simulink model "SimForcesGP2017a"  (R2020b)
settings: Solver=ode4  StartTime=0.0  StopTime=10  FixedStep=0.001  MaxStep=0.001  RelTol=1e-7
values from neighbouring files (symbols this model uses):
  B11_r_B11C = [0.23805608; 0.13201777; 0]    [InitializeSimulationGP.m]
  B11_r_B11Tc1 = [L11; 0; 0]    [InitializeSimulationGP.m]
  B11_Rot_Tc1 = eye(3)    [InitializeSimulationGP.m]
  B11cI = [0.28426000 -0.06487287 0;         -0.06487287  0.54237481 0;                   0  0          0.67891020]    [InitializeSimulationGP.m]
  B12_r_B12C = [0.60504569; 0.27199376; 0.00002484]    [InitializeSimulationGP.m]
  B12_r_B12Tc2 = [L21;0;0]    [InitializeSimulationGP.m]
  B12_Rot_Tc2 = eye(3)    [InitializeSimulationGP.m]
  B12cI = [1.18803886 -2.36786418 0.00280315;          -2.36786418 6.31493281 0.00022322;           0.00280315 0.00022322 7.40915161]    [InitializeSimulationGP.m]
  B31_r_B31C = [0.35781210 0 0]    [InitializeSimulationGP.m]
  B31_Rot_B41 = eye(3)    [InitializeSimulationGP.m]
  B31cI = diag([0.03150902 0.90735702 0.90763033])    [InitializeSimulationGP.m]
  B32_r_B32C = [0.35781210 0 0]    [InitializeSimulationGP.m]
  B32_Rot_B42 = eye(3)    [InitializeSimulationGP.m]
  B32cI = diag([0.03150902 0.90735702 0.90763033])    [InitializeSimulationGP.m]
  B41_r_B41C = [0.55785997 0 0]    [InitializeSimulationGP.m]
  B41_r_B41Tc1 = [lc1;0;0]    [InitializeSimulationGP.m]
  B41cI = diag([0.00370720 0.55759812 0.55785997])    [InitializeSimulationGP.m]
  B42_r_B42C = [0.55785997 0 0]    [InitializeSimulationGP.m]
  B42_r_B42Tc2 = [lc2; 0; 0]    [InitializeSimulationGP.m]
  B42cI = diag([0.00370720 0.55759812 0.55785997])    [InitializeSimulationGP.m]
  B52_r_B52C = [0 0 0.56802906]    [InitializeSimulationGP.m]
  B52_r_B52P32 = [lc3; 0; 0]    [InitializeSimulationGP.m]
  B52_Rot_P32 = eye(3)    [InitializeSimulationGP.m]
  B52cI = diag([0.91789884, 0.91790043, 0.00091463])    [InitializeSimulationGP.m]
  Bc1_r_Bc1B11 = [L1; 0; 0]    [InitializeSimulationGP.m]
  Bc1_r_Bc1B31 = [0;0;0]    [InitializeSimulationGP.m]
  Bc1_r_Bc1C = [0.14178771; 0.16555780; 0]    [InitializeSimulationGP.m]
  Bc1_V = [0;0;0;0;0;0]    [InitializeSimulationGP.m]
  Bc1cI = [+5.892211080 +5.476111360 -0.000019630;          +5.476111360 +28.66965601 -0.000024550;          -0.000019630 -0.000024550 +29.78955950]    [InitializeSimulationGP.m]
  Bc2_r_Bc2B12 = [L2;0;0]    [InitializeSimulationGP.m]
  Bc2_r_Bc2B32 = [0;0;0]    [InitializeSimulationGP.m]
  Bc2_r_Bc2C = [0.54319901; 0.10543875; 0]    [InitializeSimulationGP.m]
  Bc2cI = [0.48071390 0.52924041 0;          0.52924041 5.80912352 0;              0      0          5.97255351]    [InitializeSimulationGP.m]
  beta1 = atan2d(374.261,935)*pi/180    [InitializeSimulationGP.m]
  beta2 = atan2d(45.757,373.313)*pi/180    [InitializeSimulationGP.m]
  beta3 = atan2d(139.50,1132.19)*pi/180    [InitializeSimulationGP.m]
  beta4 = atan2d(88.061,296.198)*pi/180    [InitializeSimulationGP.m]
  D22F = [0;0;0;0;0;0]    [InitializeSimulationGP.m]
  L1 = 1.0071227324212    (= 1.00712273242)    [InitializeSimulationGP.m]
  L11 = 0.37610632101293    (= 0.376106321013)    [InitializeSimulationGP.m]
  L2 = 1.132185817991    (= 1.13218581799)    [InitializeSimulationGP.m]
  L21 = 0.30901132665325    (= 0.309011326653)    [InitializeSimulationGP.m]
  lc1 = 0.745    [InitializeSimulationGP.m]
  lc2 = 0.745    [InitializeSimulationGP.m]
  mB11 = 25.52660174    [InitializeSimulationGP.m]
  mB12 = 33.92850233    [InitializeSimulationGP.m]
  mB31 = 17.36281648    [InitializeSimulationGP.m]
  mB32 = 17.36281648    [InitializeSimulationGP.m]
  mB41 = 10.34519231    [InitializeSimulationGP.m]
  mB42 = 10.34519231    [InitializeSimulationGP.m]
  mB52 = 6.73059863    [InitializeSimulationGP.m]
  mBc1 = 307.29601379    [InitializeSimulationGP.m]
  mBc2 = 54.58702836    [InitializeSimulationGP.m]
  mP22 = 9.26136143    [InitializeSimulationGP.m]
  mP32 = 570.18877059    [InitializeSimulationGP.m]
  P22_r_P22C = [0.62192523 0 0]    [InitializeSimulationGP.m]
  P22_Rot_B52 = eye(3)    [InitializeSimulationGP.m]
  P22cI = diag([0.00662754, 1.48387017, 1.48398069])    [InitializeSimulationGP.m]
  P32_r_P32C = [0.25466704; -0.13034397; -0.01302248]    [InitializeSimulationGP.m]
  P32_r_P32D22 = [0.40499744871392; -0.13130517281345; -0.013385243295654]    [InitializeSimulationGP.m]
  P32_Rot_D22 = [1 0 0;              0 0.9707729441837 0.23999977258512;              0 -0.23999977258512 0.9707729441837]    [InitializeSimulationGP.m]
  P32cI = [46.81220713 0.38607676 -0.00453819;          0.38607676 71.92201786 -1.14320993;          -0.00453819 -1.14320993 67.38128576]    [InitializeSimulationGP.m]
  Tc1_r_Tc1Bc2 = [0.098495302558553; 0.01838181329939; 0]    [InitializeSimulationGP.m]
  Tc1_Rot_Bc2 = [cos(alpha2) -sin(alpha2) 0;                sin(alpha2)  cos(alpha2) 0;                0            0           1]    [InitializeSimulationGP.m]
  Tc2_r_Tc2P22 = [-0.048858374920227;0.36587359346146;0.035276938723102]    [InitializeSimulationGP.m]
  Tc2_Rot_P22 = [0.95853460763586 -0.27664713597974  0.0683942111482;                0.28497614981675  0.93051946315663 -0.23004808784757;                0                 0.23999977258511  0.9707729441837]    [InitializeSimulationGP.m]
  Th1A = 5*pi/180    (= 0.0872664625997)    [InitializeSimulationGP.m]
  Th1B = 20*pi/180    (= 0.349065850399)    [InitializeSimulationGP.m]
  Th1f = 1    [InitializeSimulationGP.m]
  Th2A = 15*pi/180    (= 0.261799387799)    [InitializeSimulationGP.m]
  Th2B = -50*pi/180    (= -0.872664625997)    [InitializeSimulationGP.m]
  Th2f = 2    [InitializeSimulationGP.m]
  W_r_WBc1 = [0.185;-0.085;0]    [InitializeSimulationGP.m]
  W_Rot_Bc1 = [cos(alpha1) -sin(alpha1) 0;              sin(alpha1)  cos(alpha1) 0;              0            0           1]    [InitializeSimulationGP.m]
  Wg = [0; 9.8066; 0]    [InitializeSimulationGP.m]
  x10 = 0.83    [InitializeSimulationGP.m]
  x20 = 0.83    [InitializeSimulationGP.m]
  xf = [1;0;0;0;0;0]    [InitializeSimulationGP.m]
  xt2A = 0.1    [InitializeSimulationGP.m]
  xt2B = 0.5    [InitializeSimulationGP.m]
  xt2f = 1    [InitializeSimulationGP.m]
  ztau = [0;0;0;0;0;1]    [InitializeSimulationGP.m]
undefined symbols (not defined in the file or in its folder): B11_V, B11_V_SS, B11Ftot, B12_U_Tc2, B12_V, B12_V_SS, B12Ftot, B31_r_B31B41, B31_V, B31_V_SS, B31FTot, B32_r_B32B42, B32_U_B42, B32_V, B32_V_SS, B32FTot, B41_V, B41_V_SS, B41FTot, B42_Rot_Tc2, B42_U_Tc2, B42_V, B42_V_SS, B42FTot, B52_U_P32, B52_V, B52_V_SS, B52Ftot, Bc1_V_SS, Bc1Tot, Bc2_Rot_B12, Bc2_Rot_B32, Bc2_U_B12, Bc2_U_B32, Bc2_V, Bc2_V_SS, Bc2Tot, D22_V, D22_V_SS, dq1, dq11, dq12, dq2, dq21, dq22, dx1, dx2, FTot_S1, FTot_S2P, FTot_S2R, P22_r_P22B52, P22_U_B52, P22_V, P22_V_SS, P22FTot, P32_U_D22, P32_V, P32_V_SS, P32FTot, q1 ... (+28)
libraries: nesl_utility x94, sm_lib x45
(part 3 of 5)

== system SimForcesGP2017a/Hydraulic manipulator, Simscape/TiltCylinderAndTiltPiston ==
  B32Aux : sm_lib/Frames and Transforms/Rigid Transform  TranslationMethod=None  TranslationStandardOffset=0  TranslationLengthUnit=m  TranslationStandardAxis=+Z  TranslationCartesianOffset=[0 0 0]  TranslationROffset=0  TranslationROffsetUnits=m  TranslationZOffset=0  TranslationZOffsetUnits=m  TranslationThetaOffset=0  TranslationThetaOffsetUnits=deg  RotationMethod=StandardAxis  RotationAngleUnits=deg  RotationStandardAxis=+Y  RotationAngle=90  RotationArbitraryAxis=[0 0 1]  FollAlignAxisA=+X  BaseAlignAxisA=+Y  FollAlignAxisB=+Y  BaseAlignAxisB=+Z  RotationSequenceAxes=FollowerAxes  RotationSequence=XYX  RotationSequenceAngles=[0 0 0]  RotationSequenceAnglesUnits=deg  RotationMatrix=[1 0 0; 0 1 0; 0 0 1]
  B42Aux : sm_lib/Frames and Transforms/Rigid Transform  TranslationMethod=None  TranslationStandardOffset=0  TranslationLengthUnit=m  TranslationStandardAxis=+Z  TranslationCartesianOffset=[0 0 0]  TranslationROffset=0  TranslationROffsetUnits=m  TranslationZOffset=0  TranslationZOffsetUnits=m  TranslationThetaOffset=0  TranslationThetaOffsetUnits=deg  RotationMethod=StandardAxis  RotationAngleUnits=deg  RotationStandardAxis=+Y  RotationAngle=-90  RotationArbitraryAxis=[0 0 1]  FollAlignAxisA=+X  BaseAlignAxisA=+Y  FollAlignAxisB=+Y  BaseAlignAxisB=+Z  RotationSequenceAxes=FollowerAxes  RotationSequence=XYX  RotationSequenceAngles=[0 0 0]  RotationSequenceAnglesUnits=deg  RotationMatrix=[1 0 0; 0 1 0; 0 0 1]
  PS-Sim2 : nesl_utility/PS-Simulink Converter  PhysicalDomain=network_engine_domain  SubClassName=ps_output  LeftPortType=input  RightPortType=output  PseudoPeriodic=off  Frequencies=[]  Unit=inherit  AffineConversion=off
  Tilt cylinder rotation (q21) : sm_lib/Joints/Revolute Joint  JointMode=Normal  SenseConstraintForce=off  SenseConstraintForceX=off  SenseConstraintForceY=off  SenseConstraintForceZ=off  SenseConstraintTorque=off  SenseConstraintTorqueX=off  SenseConstraintTorqueY=off  SenseConstraintTorqueZ=off  SenseTotalForce=off  SenseTotalForceX=off  SenseTotalForceY=off  SenseTotalForceZ=off  SenseTotalTorque=off  SenseTotalTorqueX=off  SenseTotalTorqueY=off  SenseTotalTorqueZ=off  CompositeWrenchDir=FollowerOnBase  CompositeWrenchFrame=BaseFrame  EquilibriumPosition=0  EquilibriumPositionUnits=deg  SpringStiffness=0  SpringStiffnessUnits=N*m/deg  DampingCoefficient=0  DampingCoefficientUnits=N*m/(deg/s)  TorqueActuationMode=NoTorque  MotionActuationMode=ComputedMotion  SensePosition=off  SenseVelocity=off  SenseAcceleration=off  SenseTorqueForce=off  SenseLowerLimitTorqueForce=off  SenseUpperLimitTorqueForce=off  LowerLimitSpecify=off  LowerLimitBound=-90  LowerLimitBoundUnits=deg  LowerLimitStiffness=1e4  LowerLimitStiffnessUnits=N*m/deg  LowerLimitDamping=10  LowerLimitDampingUnits=N*m/(deg/s)  LowerLimitTransitionRegionWidth=0.1  LowerLimitTransitionRegionWidthUnits=deg  UpperLimitSpecify=off  UpperLimitBound=90  UpperLimitBoundUnits=deg  UpperLimitStiffness=1e4  UpperLimitStiffnessUnits=N*m/deg  UpperLimitDamping=10  UpperLimitDampingUnits=N*m/(deg/s)  UpperLimitTransitionRegionWidth=0.1  UpperLimitTransitionRegionWidthUnits=deg  PositionTargetSpecify=off  PositionTargetPriority=High  PositionTargetValue=0  PositionTargetValueUnits=deg  VelocityTargetSpecify=off  VelocityTargetPriority=High  VelocityTargetValue=0  VelocityTargetValueUnits=deg/s
  Tilt piston rotation (q22) : sm_lib/Joints/Revolute Joint  JointMode=Normal  SenseConstraintForce=off  SenseConstraintForceX=off  SenseConstraintForceY=off  SenseConstraintForceZ=off  SenseConstraintTorque=off  SenseConstraintTorqueX=off  SenseConstraintTorqueY=off  SenseConstraintTorqueZ=off  SenseTotalForce=off  SenseTotalForceX=off  SenseTotalForceY=off  SenseTotalForceZ=off  SenseTotalTorque=off  SenseTotalTorqueX=off  SenseTotalTorqueY=off  SenseTotalTorqueZ=off  CompositeWrenchDir=FollowerOnBase  CompositeWrenchFrame=BaseFrame  EquilibriumPosition=0  EquilibriumPositionUnits=deg  SpringStiffness=0  SpringStiffnessUnits=N*m/deg  DampingCoefficient=0  DampingCoefficientUnits=N*m/(deg/s)  TorqueActuationMode=NoTorque  MotionActuationMode=ComputedMotion  SensePosition=off  SenseVelocity=off  SenseAcceleration=off  SenseTorqueForce=off  SenseLowerLimitTorqueForce=off  SenseUpperLimitTorqueForce=off  LowerLimitSpecify=off  LowerLimitBound=-90  LowerLimitBoundUnits=deg  LowerLimitStiffness=1e4  LowerLimitStiffnessUnits=N*m/deg  LowerLimitDamping=10  LowerLimitDampingUnits=N*m/(deg/s)  LowerLimitTransitionRegionWidth=0.1  LowerLimitTransitionRegionWidthUnits=deg  UpperLimitSpecify=off  UpperLimitBound=90  UpperLimitBoundUnits=deg  UpperLimitStiffness=1e4  UpperLimitStiffnessUnits=N*m/deg  UpperLimitDamping=10  UpperLimitDampingUnits=N*m/(deg/s)  UpperLimitTransitionRegionWidth=0.1  UpperLimitTransitionRegionWidthUnits=deg  PositionTargetSpecify=off  PositionTargetPriority=High  PositionTargetValue=0  PositionTargetValueUnits=deg  VelocityTargetSpecify=off  VelocityTargetPriority=High  VelocityTargetValue=0  VelocityTargetValueUnits=deg/s
  TiltCylinderSolid : sm_lib/Body Elements/File Solid  ExtGeomFileName=05_TiltCylGP.STEP  UnitType=FromFile  ExtGeomFileUnits=m  StepReaderType=OCC  ExportConvexHullGeometry=off  InertiaType=Custom  Mass=17.36281648  MassUnits=kg  CenterOfMass=[0 0.31781210 0]  CenterOfMassUnits=m  MomentsOfInertia=[0.90735702 0.03150902 0.90763033]  MomentsOfInertiaUnits=kg*m^2  ProductsOfInertia=[0 0 0]  ProductsOfInertiaUnits=kg*m^2  BasedOnType=Density  Density=7300  DensityUnits=kg/m^3  DoExposeReferenceFrame=off  SerializedFrames=<Frames><Frame><Id>Frame1</Id><Value><Name>B32</Name><Origin><Source>GeometricFeature</Source><FeatureName>cylindrical surface 11</FeatureName></Origin><PrimaryAxis><DefinedDirection>+X</DefinedDirection><Source>ReferenceFrame</Source><SourceDirection>+Y</SourceDirection><FeatureName></FeatureName></PrimaryAxis><SecondaryAxis><DefinedDirection>+Y</DefinedDirection><Source>ReferenceFrame</Source><SourceDirection>-X</SourceDirection><FeatureName></FeatureName></SecondaryAxis></Value></Frame><Frame><Id>Frame2</Id><Value><Name>B32Aux</Name><Origin><Source>GeometricFeature</Source><FeatureName>planar surface 4</FeatureName></Origin><PrimaryAxis><DefinedDirection>+X</DefinedDirection><Source>ReferenceFrame</Source><SourceDirection>+Y</SourceDirection><FeatureName></FeatureName></PrimaryAxis><SecondaryAxis><DefinedDirection>+Y</DefinedDirection><Source>ReferenceFrame</Source><SourceDirection>-X</SourceDirection><FeatureName></FeatureName></SecondaryAxis></Value></Frame></Frames>  GraphicType=FromGeometry  MarkerShape=Sphere  MarkerSize=10  GraphicVisPropType=SimpleVisualProperties  GraphicDiffuseColor=[1 1 119]/255  GraphicSpecularColor=[0.5 0.5 0.5 1.0]  GraphicAmbientColor=[0.15 0.15 0.15 1.0]  GraphicEmissiveColor=[0.0 0.0 0.0 1.0]  GraphicShininess=75  GraphicOpacity=1.0
  TiltPistonSolid : sm_lib/Body Elements/File Solid  ExtGeomFileName=06_TiltPistGP.STEP  UnitType=FromFile  ExtGeomFileUnits=m  StepReaderType=OCC  ExportConvexHullGeometry=off  InertiaType=Custom  Mass=10.34519231  MassUnits=kg  CenterOfMass=[0 0.32981882 0]  CenterOfMassUnits=m  MomentsOfInertia=[0.55759812 0.00370720 0.55785997]  MomentsOfInertiaUnits=kg*m^2  ProductsOfInertia=[0 0 0]  ProductsOfInertiaUnits=kg*m^2  BasedOnType=Density  Density=7850  DensityUnits=kg/m^3  DoExposeReferenceFrame=off  SerializedFrames=<Frames><Frame><Id>Frame2</Id><Value><Name>B42</Name><Origin><Source>GeometricFeature</Source><FeatureName>planar surface 2</FeatureName></Origin><PrimaryAxis><DefinedDirection>+X</DefinedDirection><Source>ReferenceFrame</Source><SourceDirection>+Y</SourceDirection><FeatureName></FeatureName></PrimaryAxis><SecondaryAxis><DefinedDirection>+Y</DefinedDirection><Source>ReferenceFrame</Source><SourceDirection>-X</SourceDirection><FeatureName></FeatureName></SecondaryAxis></Value></Frame><Frame><Id>Frame3</Id><Value><Name>P11</Name><Origin><Source>GeometricFeature</Source><FeatureName>cylindrical surface 8</FeatureName></Origin><PrimaryAxis><DefinedDirection>+X</DefinedDirection><Source>ReferenceFrame</Source><SourceDirection>+Y</SourceDirection><FeatureName></FeatureName></PrimaryAxis><SecondaryAxis><DefinedDirection>+Y</DefinedDirection><Source>ReferenceFrame</Source><SourceDirection>-X</SourceDirection><FeatureName></FeatureName></SecondaryAxis></Value></Frame></Frames>  GraphicType=FromGeometry  MarkerShape=Sphere  MarkerSize=10  GraphicVisPropType=SimpleVisualProperties  GraphicDiffuseColor=[9 232 232]/255  GraphicSpecularColor=[0.5 0.5 0.5 1.0]  GraphicAmbientColor=[0.15 0.15 0.15 1.0]  GraphicEmissiveColor=[0.0 0.0 0.0 1.0]  GraphicShininess=75  GraphicOpacity=1.0
  x2-translation : sm_lib/Joints/Prismatic Joint  JointMode=Normal  SenseConstraintForce=off  SenseConstraintForceX=off  SenseConstraintForceY=off  SenseConstraintForceZ=off  SenseConstraintTorque=off  SenseConstraintTorqueX=off  SenseConstraintTorqueY=off  SenseConstraintTorqueZ=off  SenseTotalForce=off  SenseTotalForceX=off  SenseTotalForceY=off  SenseTotalForceZ=off  SenseTotalTorque=off  SenseTotalTorqueX=off  SenseTotalTorqueY=off  SenseTotalTorqueZ=off  CompositeWrenchDir=FollowerOnBase  CompositeWrenchFrame=FollowerFrame  EquilibriumPosition=0  EquilibriumPositionUnits=m  SpringStiffness=0  SpringStiffnessUnits=N/m  DampingCoefficient=0  DampingCoefficientUnits=N/(m/s)  TorqueActuationMode=ComputedTorque  MotionActuationMode=ComputedMotion  SensePosition=off  SenseVelocity=off  SenseAcceleration=off  SenseTorqueForce=on  SenseLowerLimitTorqueForce=off  SenseUpperLimitTorqueForce=off  LowerLimitSpecify=off  LowerLimitBound=-1  LowerLimitBoundUnits=m  LowerLimitStiffness=1e6  LowerLimitStiffnessUnits=N/m  LowerLimitDamping=1e3  LowerLimitDampingUnits=N/(m/s)  LowerLimitTransitionRegionWidth=1e-4  LowerLimitTransitionRegionWidthUnits=m  UpperLimitSpecify=off  UpperLimitBound=1  UpperLimitBoundUnits=m  UpperLimitStiffness=1e6  UpperLimitStiffnessUnits=N/m  UpperLimitDamping=1e3  UpperLimitDampingUnits=N/(m/s)  UpperLimitTransitionRegionWidth=1e-4  UpperLimitTransitionRegionWidthUnits=m  PositionTargetSpecify=on  PositionTargetPriority=Low  PositionTargetValue=0.4  PositionTargetValueUnits=m  VelocityTargetSpecify=off  VelocityTargetPriority=High  VelocityTargetValue=0  VelocityTargetValueUnits=m/s
  B32 : PMIOPort  Side=Left
  B42 : PMIOPort  Port=2  Side=Left
  F4 : PMIOPort  Port=3  Side=Right
  F6 : PMIOPort  Port=4  Side=Right
  fc2 : Outport
  wires:
  PS-Sim2/1 -> fc2/1
  connections:
  TiltCylinderSolid/RConn1 -- B32Aux/LConn1
  x2-translation/RConn1 -- B42Aux/LConn1
  Tilt cylinder rotation (q21)/RConn1 -- TiltCylinderSolid/LConn1 -- B32/RConn1
  B42/RConn1 -- TiltPistonSolid/LConn1 -- B42Aux/RConn1
  B32Aux/RConn1 -- x2-translation/LConn1
  Tilt cylinder rotation (q21)/LConn1 -- F4/RConn1
  TiltPistonSolid/RConn1 -- Tilt piston rotation (q22)/LConn1
  Tilt piston rotation (q22)/RConn1 -- F6/RConn1
  PS-Sim2/LConn1 -- x2-translation/RConn2

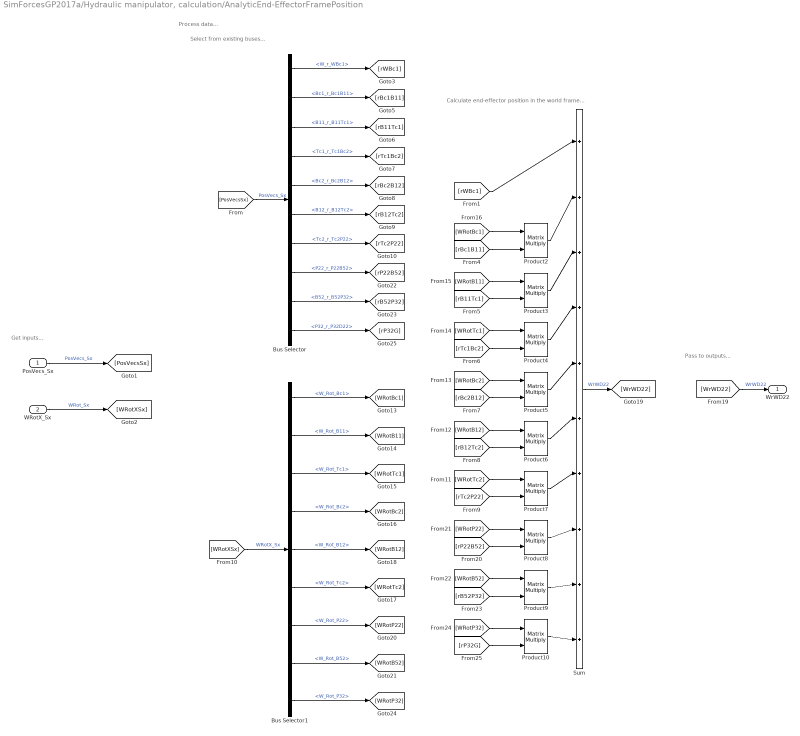
== system SimForcesGP2017a/Hydraulic manipulator, calculation/AnalyticEnd-EffectorFramePosition ==
  note: Pass to outputs...
  note: Process data...
  note: Select from existing buses...
  note: Calculate end-effector position in the world frame...
  note: Get inputs...
  PosVecs_Sx : Inport
  WRotX_Sx : Inport  Port=2
  Bus Selector : BusSelector  OutputSignals=PosVecs_S1.W_r_WBc1,PosVecs_S1.Bc1_r_Bc1B11,PosVecs_S1.B11_r_B11Tc1,PosVecs_S1.Tc1_r_Tc1Bc2,PosVecs_S2R.Bc2_r_Bc2B12,PosVecs_S2R.B12_r_B12Tc2,PosVecs_S2R.Tc2_r_Tc2P22,PosVecs_S2P.P22_r_P22B52,PosVecs_S2P.B52_r_B52P32,PosVecs_S2P.P32_r_P32D22
  Bus Selector1 : BusSelector  OutputSignals=WRotX_S1.W_Rot_Bc1,WRotX_S1.W_Rot_B11,WRotX_S1.W_Rot_Tc1,WRotX_S1.W_Rot_Bc2,WRotX_S2R.W_Rot_B12,WRotX_S2R.W_Rot_Tc2,WRotX_S2R.W_Rot_P22,WRotX_S2P.W_Rot_B52,WRotX_S2P.W_Rot_P32
  Product{2..10} (9 alike) : Product  Multiplication=Matrix(*)
  Sum : Sum  Inputs=|++++++++++
  WrWD22 : Outport
  wires:
  WRotX_Sx/1 -> [WRotXSx]  "WRot_Sx"
  PosVecs_Sx/1 -> [PosVecsSx]  "PosVecs_Sx"
  [PosVecsSx] -> Bus Selector/1  "PosVecs_Sx"
  Bus Selector/2 -> [rBc1B11]  "<Bc1_r_Bc1B11>"
  Bus Selector/3 -> [rB11Tc1]  "<B11_r_B11Tc1>"
  Bus Selector/7 -> [rTc2P22]  "<Tc2_r_Tc2P22>"
  Bus Selector/6 -> [rB12Tc2]  "<B12_r_B12Tc2>"
  Bus Selector/5 -> [rBc2B12]  "<Bc2_r_Bc2B12>"
  Bus Selector/4 -> [rTc1Bc2]  "<Tc1_r_Tc1Bc2>"
  [rBc1B11] -> Product2/2
  [rB11Tc1] -> Product3/2
  [rTc1Bc2] -> Product4/2
  [rBc2B12] -> Product5/2
  [rB12Tc2] -> Product6/2
  [rTc2P22] -> Product7/2
  [WRotXSx] -> Bus Selector1/1  "WRotX_Sx"
  Bus Selector1/1 -> [WRotBc1]  "<W_Rot_Bc1>"
  Bus Selector1/2 -> [WRotB11]  "<W_Rot_B11>"
  Bus Selector1/3 -> [WRotTc1]  "<W_Rot_Tc1>"
  Bus Selector1/4 -> [WRotBc2]  "<W_Rot_Bc2>"
  Bus Selector1/5 -> [WRotB12]  "<W_Rot_B12>"
  Bus Selector1/6 -> [WRotTc2]  "<W_Rot_Tc2>"
  [WRotTc2] -> Product7/1
  [WRotB12] -> Product6/1
  [WRotBc2] -> Product5/1
  [WRotTc1] -> Product4/1
  [WRotB11] -> Product3/1
  [WRotBc1] -> Product2/1
  Sum/1 -> [WrWD22]  "WrWD22"
  [WrWD22] -> WrWD22/1  "WrWD22"
  Bus Selector1/7 -> [WRotP22]  "<W_Rot_P22>"
  Bus Selector1/8 -> [WRotB52]  "<W_Rot_B52>"
  Bus Selector/8 -> [rP22B52]  "<P22_r_P22B52>"
  Bus Selector/9 -> [rB52P32]  "<B52_r_B52P32>"
  [rP22B52] -> Product8/2
  [WRotP22] -> Product8/1
  [WRotB52] -> Product9/1
  [rB52P32] -> Product9/2
  Bus Selector1/9 -> [WRotP32]  "<W_Rot_P32>"
  Bus Selector/10 -> [rP32G]  "<P32_r_P32D22>"
  [rP32G] -> Product10/2
  [WRotP32] -> Product10/1
  Bus Selector/1 -> [rWBc1]  "<W_r_WBc1>"
  [rWBc1] -> Sum/1
  Product2/1 -> Sum/2
  Product3/1 -> Sum/3
  Product4/1 -> Sum/4
  Product5/1 -> Sum/5
  Product6/1 -> Sum/6
  Product7/1 -> Sum/7
  Product8/1 -> Sum/8
  Product9/1 -> Sum/9
  Product10/1 -> Sum/10

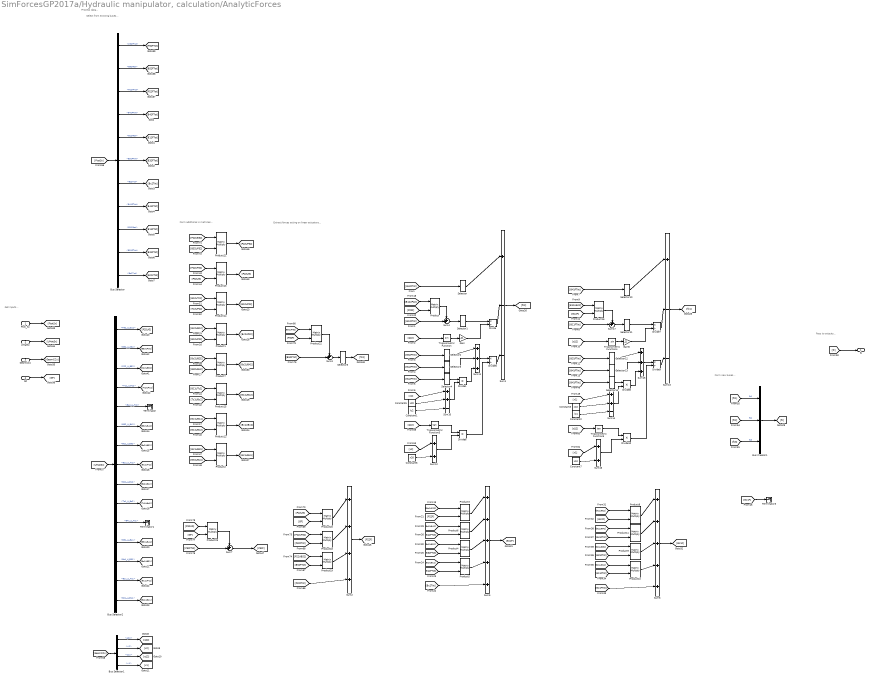
== system SimForcesGP2017a/Hydraulic manipulator, calculation/AnalyticForces ==
  note: Pass to outputs...
  note: Form new buses...
  note: Process data...
  note: Extract forces acting on linear actuators...
  note: Form additional U matrices...
  note: Select from existing buses...
  note: Get inputs...
  Ftot_Sx : Inport
  UMatSx : Inport  Port=2
  GeomCCx : Inport  Port=3
  GF : Inport  Port=4
  Bus Creator1 : BusCreator  Inputs=3
  Bus Selector : BusSelector  OutputSignals=FTot_S2P.P32FTot,FTot_S2P.B52Ftot,FTot_S2P.P22FTot,FTot_S2R.B42FTot,FTot_S2R.B12Ftot,FTot_S2R.B32FTot,FTot_S2R.Bc2Tot,FTot_S1.B41FTot,FTot_S1.B11Ftot,FTot_S1.B31FTot,FTot_S1.Bc1Tot
  Bus Selector1 : BusSelector  OutputSignals=Geom_S2R.q22,Geom_S2R.x2,Geom_S1.q12,Geom_S1.x1
  Bus Selector2 : BusSelector  OutputSignals=UMats_S2P.P32_U_D22,UMats_S2P.B52_U_P32,UMats_S2P.P22_U_B52,UMats_S2R.Tc2_U_P22,UMats_S2R.B42_U_Tc2,UMats_S2R.B32_U_B42,UMats_S2R.Bc2_U_B32,UMats_S2R.B12_U_Tc2,UMats_S2R.Bc2_U_B12,UMats_S1.Tc1_U_Bc2,UMats_S1.B41_U_Tc1,UMats_S1.B31_U_B41,UMats_S1.Bc1_U_B31,UMats_S1.B11_U_Tc1,UMats_S1.Bc1_U_B11
  Constant1 : Constant  Value=lc2
  Constant2 : Constant  Value=lc1
  Constant3 : Constant  Value=x10
  Constant5 : Constant  Value=x20
  Constant6 : Constant  Value=x20
  Constant7 : Constant  Value=x10
  Divide{,5,7,9} (4 alike) : Product  Inputs=*/
  Divide{1,6,8,10} (4 alike) : Product  Inputs=**
  Gain : Gain  Gain=L21
  Gain5 : Gain  Gain=L11
  Product{,1..16,18..23} (23 alike) : Product  Multiplication=Matrix(*)
  Selector : Selector  InputPortWidth=6  IndexOptions=Index vector (dialog)  Indices=[1]  OutputSizes=1
  Selector{1..3,11..13} (6 alike) : Selector  InputPortWidth=6  IndexOptions=Index vector (dialog)  Indices=[6]  OutputSizes=1
  Selector10 : Selector  InputPortWidth=6  IndexOptions=Index vector (dialog)  Indices=[1]  OutputSizes=1
  Selector14 : Selector  InputPortWidth=6  IndexOptions=Index vector (dialog)  Indices=[2]  OutputSizes=1
  Selector4 : Selector  InputPortWidth=6  IndexOptions=Index vector (dialog)  Indices=[2]  OutputSizes=1
  Selector5 : Selector  InputPortWidth=6  IndexOptions=Index vector (dialog)  Indices=[1]  OutputSizes=1
  Sum1 : Sum  Inputs=|+--
  Sum10 : Sum  Inputs=|++-
  Sum11 : Sum  Inputs=|+++
  Sum12 : Sum  Inputs=|++
  Sum13 : Sum  Inputs=|+--
  Sum14 : Sum  Inputs=|++-
  Sum15 : Sum  Inputs=|+++
  Sum16 : Sum  Inputs=|++
  Sum{3..4,7,17} (4 alike) : Sum  Inputs=++|
  Sum2 : Sum  Inputs=|++++
  Sum5 : Sum  Inputs=|+++++
  Sum6 : Sum  Inputs=|+++++
  Terminator : Terminator
  Terminator1 : Terminator
  Terminator3 : Terminator
  Trigonometric Function : Trigonometry
  Trigonometric Function3 : Trigonometry  Operator=tan
  Trigonometric Function4 : Trigonometry
  Trigonometric Function5 : Trigonometry  Operator=tan
  fc : Outport
  wires:
  Bus Selector/4 -> [B42FTot]  "<B42FTot>"
  Bus Selector/6 -> [B32FTot]  "<B32FTot>"
  Bus Selector/5 -> [B12FTot]  "<B12Ftot>"
  Bus Selector/7 -> [Bc2Tot]  "<Bc2Tot>"
  Bus Selector/8 -> [B41FTot]  "<B41FTot>"
  Bus Selector/9 -> [B11FTot]  "<B11Ftot>"
  Bus Selector/10 -> [B31FTot]  "<B31FTot>"
  Bus Selector/11 -> [Bc1FTot]  "<Bc1Tot>"
  [B42FTot] -> Selector/1
  Bus Selector1/1 -> [q22]  "<q22>"
  Bus Selector1/2 -> [x2]  "<x2>"
  Bus Selector1/4 -> [x1]  "<x1>"
  Bus Selector1/3 -> [q12]  "<q12>"
  Gain/1 -> Divide/2
  Trigonometric Function/1 -> Gain/1
  Selector/1 -> Sum1/1
  Divide/1 -> Sum1/2
  Sum1/1 -> [fc2]
  Bus Selector2/4 -> [Tc2UP22]  "<Tc2_U_P22>"
  Bus Selector2/5 -> Terminator/1  "<B42_U_Tc2>"
  Bus Selector2/6 -> [B32UB42]  "<B32_U_B42>"
  Bus Selector2/7 -> [Bc2UB32]  "<Bc2_U_B32>"
  Bus Selector2/8 -> [B12UTc2]  "<B12_U_Tc2>"
  Bus Selector2/9 -> [Bc2UB12]  "<Bc2_U_B12>"
  Bus Selector2/10 -> [Tc1UBc2]  "<Tc1_U_Bc2>"
  Bus Selector2/11 -> Terminator1/1  "<B41_U_Tc1>"
  Bus Selector2/12 -> [B31UB41]  "<B31_U_B41>"
  Bus Selector2/13 -> [Bc1UB31]  "<Bc1_U_B31>"
  Bus Selector2/14 -> [B11UTc1]  "<B11_U_Tc1>"
  Bus Selector2/15 -> [Bc1UB11]  "<Bc1_U_B11>"
  [B12FTot] -> Sum4/2
  Product/1 -> Sum4/1
  Sum4/1 -> Selector1/1
  [B12UP22] -> Product/1
  [Bc2UP22] -> Product3/1
  [P22F] -> Product/2
  [P22F] -> Product3/2
  Product3/1 -> Sum5/1
  [Bc2Tot] -> Sum5/5
  Product6/1 -> Sum5/2
  Product4/1 -> Sum5/3
  Product5/1 -> Sum5/4
  [B12FTot] -> Product5/2
  [Bc2UB12] -> Product5/1
  [B32FTot] -> Product4/2
  [B42FTot] -> Product6/2
  [B32UB42] -> Product7/2
  [Bc2UB32] -> Product7/1
  Product7/1 -> [Bc2UB42]
  [Bc2UB42] -> Product6/1
  [Bc2UB32] -> Product4/1
  Sum5/1 -> [Bc2F]
  Sum6/1 -> [Bc1F]
  [Bc1UB31] -> Product9/1
  [Bc1UB41] -> Product11/1
  [B41FTot] -> Product11/2
  [B31FTot] -> Product9/2
  [Bc1UB11] -> Product10/1
  [B11FTot] -> Product10/2
  Product10/1 -> Sum6/4
  Product9/1 -> Sum6/3
  Product11/1 -> Sum6/2
  [Bc1FTot] -> Sum6/5
  Product8/1 -> Sum6/1
  [Bc2F] -> Product8/2
  [Bc1UBc2] -> Product8/1
  Product1/1 -> [Bc2UP22]
  Product2/1 -> [Bc1UB41]
  [Bc1UB31] -> Product2/1
  [B31UB41] -> Product2/2
  [B12UTc2] -> Product14/1
  [Tc2UP22] -> Product14/2
  Product14/1 -> [B12UP22]
  [B12UP22] -> Product1/2
  [Bc2UB12] -> Product1/1
  [Bc1UB11] -> Product12/1
  [B11UBc2] -> Product12/2
  Product15/1 -> [B11UBc2]
  [Tc1UBc2] -> Product15/2
  [B11UTc1] -> Product15/1
  Product12/1 -> [Bc1UBc2]
  Selector1/1 -> Divide/1
  Divide5/1 -> Sum1/3
  Constant6/1 -> Sum12/2
  [x2] -> Sum12/1
  Selector2/1 -> Sum11/1
  Selector3/1 -> Sum11/2
  Divide1/1 -> Sum11/3
  [B32FTot] -> Selector2/1
  [B42FTot] -> Selector3/1
  [B42FTot] -> Selector4/1
  Selector4/1 -> Divide1/1
  Sum10/1 -> Divide1/2
  Constant1/1 -> Sum10/3
  [x2] -> Sum10/1
  Constant5/1 -> Sum10/2
  [fc1] -> Bus Creator1/1  "fc1"
  [fc2] -> Bus Creator1/2  "fc2"
  [q22] -> Trigonometric Function/1
  Ftot_Sx/1 -> [FtotSx]
  UMatSx/1 -> [UMatSx]
  GeomCCx/1 -> [GeomCCx]
  GF/1 -> [GF]
  [FtotSx] -> Bus Selector/1
  [UMatSx] -> Bus Selector2/1
  [GeomCCx] -> Bus Selector1/1
  Trigonometric Function3/1 -> Divide6/1
  Sum12/1 -> Divide6/2
  Sum11/1 -> Divide5/1
  Divide6/1 -> Divide5/2
  [q22] -> Trigonometric Function3/1
  [q12] -> Trigonometric Function5/1
  Divide10/1 -> Divide9/2
  Sum15/1 -> Divide9/1
  Sum16/1 -> Divide10/2
  Trigonometric Function5/1 -> Divide10/1
  [q12] -> Trigonometric Function4/1
  Constant3/1 -> Sum14/2
  [x1] -> Sum14/1
  Constant2/1 -> Sum14/3
  Sum14/1 -> Divide8/2
  Selector14/1 -> Divide8/1
  [B41FTot] -> Selector14/1
  [B41FTot] -> Selector13/1
  [B31FTot] -> Selector12/1
  Divide8/1 -> Sum15/3
  Selector13/1 -> Sum15/2
  Selector12/1 -> Sum15/1
  [x1] -> Sum16/1
  Constant7/1 -> Sum16/2
  Divide9/1 -> Sum13/3
  Selector11/1 -> Divide7/1
  [Bc2F] -> Product16/2
  [B11UBc2] -> Product16/1
  Sum17/1 -> Selector11/1
  Product16/1 -> Sum17/1
  [B11FTot] -> Sum17/2
  Sum13/1 -> [fc1]
  Divide7/1 -> Sum13/2
  Selector10/1 -> Sum13/1
  Trigonometric Function4/1 -> Gain5/1
  Gain5/1 -> Divide7/2
  [B41FTot] -> Selector10/1
  Bus Creator1/1 -> [fc]
  [fc] -> fc/1
  Bus Selector/3 -> [P22FTot]  "<P22FTot>"
  Bus Selector/2 -> [B52FTot]  "<B52Ftot>"
  Bus Selector/1 -> [P32FTot]  "<P32FTot>"
  Bus Selector2/1 -> [P32UG]  "<P32_U_D22>"
  Bus Selector2/3 -> [P22UB52]  "<P22_U_B52>"
  Bus Selector2/2 -> [B52UP32]  "<B52_U_P32>"
  Sum2/1 -> [P22F]
  Product18/1 -> Sum2/2
  [P22FTot] -> Sum2/4
  Product19/1 -> Sum2/3
  Product20/1 -> Sum2/1
  [B52FTot] -> Product19/2
  [P32FTot] -> Product18/2
  [GF] -> Product20/2
  [P22UG] -> Product20/1
  [P22UB52] -> Product21/1
  [B52UP32] -> Product21/2
  Product21/1 -> [P22UP32]
  [P22UP32] -> Product18/1
  [P22UB52] -> Product19/1
  [B52FTot] -> Sum3/2
  Product22/1 -> Sum3/1
  [P32FTot] -> Sum7/2
  [GF] -> Product23/2
  [P32UG] -> Product23/1
  Product23/1 -> Sum7/1
  Sum7/1 -> [P32F]
  [P32F] -> Product22/2
  [B52UP32] -> Product22/1
  Sum3/1 -> Selector5/1
  Selector5/1 -> [fc3]
  [fc3] -> Bus Creator1/3  "fc3"
  [Bc1F] -> Terminator3/1
  Product13/1 -> [P22UG]
  [P32UG] -> Product13/2
  [P22UP32] -> Product13/1

== system SimForcesGP2017a/Hydraulic manipulator, calculation/AnalyticTotalForces ==
  note: Process data...
  note: Pass to outputs...
  note: Get inputs...
  Vels_Sx : Inport
  WRotX_Sx : Inport  Port=2
  Bus Creator : BusCreator  Inputs=FTot_S1,FTot_S2R,FTot_S2P
  Structure 1 : Subsystem
  Structure 2 (Prismatic segment) : Subsystem
  Structure 2 (Revolute segment) : Subsystem
  FTot_Sx : Outport
  wires:
  Vels_Sx/1 -> [VelsSx]
  WRotX_Sx/1 -> [WRotSx]
  [VelsSx] -> Structure 1/1(Vels_Sx)
  [VelsSx] -> Structure 2 (Revolute segment)/1(Vels_Sx)
  [WRotSx] -> Structure 1/2(WRotX_Sx)
  [WRotSx] -> Structure 2 (Revolute segment)/2(WRotX_Sx)
  Structure 2 (Revolute segment)/1(FTot_S2R) -> [FTotS2R]
  Structure 1/1(FTot_S1) -> [FTotS1]
  [FTotS2R] -> Bus Creator/2  "FTot_S2R"
  [FTotS1] -> Bus Creator/1  "FTot_S1"
  [FTotSx] -> FTot_Sx/1  "FTot_Sx"
  Bus Creator/1 -> [FTotSx]
  [WRotSx] -> Structure 2 (Prismatic segment)/2(WRotX_Sx)
  [VelsSx] -> Structure 2 (Prismatic segment)/1(Vels_Sx)
  Structure 2 (Prismatic segment)/1(FTot_S2P) -> [FTotS2P]
  [FTotS2P] -> Bus Creator/3  "FTot_S2P"

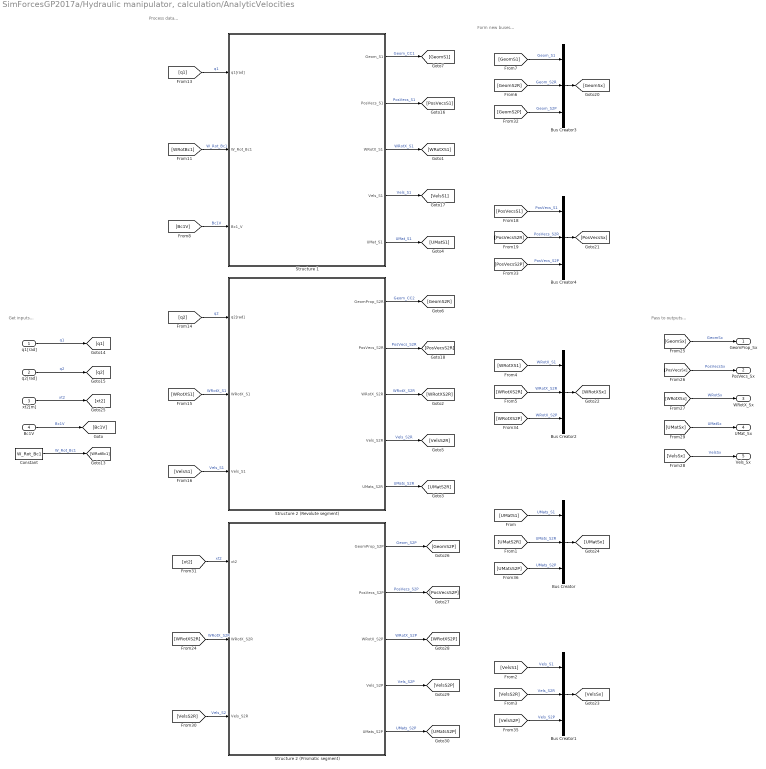
== system SimForcesGP2017a/Hydraulic manipulator, calculation/AnalyticVelocities ==
  note: Pass to outputs...
  note: Form new buses...
  note: Process data...
  note: Get inputs...
  q1[rad] : Inport  Unit=rad
  q2[rad] : Inport  Port=2
  xt2[m] : Inport  Port=3
  Bc1V : Inport  Port=4
  Bus Creator{,1..4} (5 alike) : BusCreator  Inputs=3
  Constant : Constant  Value=W_Rot_Bc1
  Structure 1 : Subsystem
  Structure 2 (Prismatic segment) : Subsystem
  Structure 2 (Revolute segment) : Subsystem
  GeomProp_Sx : Outport
  PosVecs_Sx : Outport  Port=2
  WRotX_Sx : Outport  Port=3
  UMat_Sx : Outport  Port=4
  Vels_Sx : Outport  Port=5
  wires:
  Structure 1/4(Vels_S1) -> [VelsS1]  "Vels_S1"
  [VelsS1] -> Structure 2 (Revolute segment)/3(Vels_S1)  "Vels_S1"
  Structure 2 (Revolute segment)/4(Vels_S2R) -> [VelsS2R]  "Vels_S2R"
  Structure 2 (Revolute segment)/5(UMats_S2R) -> [UMatS2R]  "UMats_S2R"
  Structure 1/5(UMat_S1) -> [UMatS1]  "UMat_S1"
  Structure 1/3(WRotX_S1) -> [WRotXS1]  "WRotX_S1"
  [WRotXS1] -> Structure 2 (Revolute segment)/2(WRotX_S1)  "WRotX_S1"
  Structure 2 (Revolute segment)/3(WRotX_S2R) -> [WRotXS2R]  "WRotX_S2R"
  Structure 2 (Revolute segment)/1(GeomProp_S2R) -> [GeomS2R]  "Geom_CC2"
  Structure 1/1(Geom_S1) -> [GeomS1]  "Geom_CC1"
  Constant/1 -> [WRotBc1]  "W_Rot_Bc1"
  [WRotBc1] -> Structure 1/2(W_Rot_Bc1)  "W_Rot_Bc1"
  [Bc1V] -> Structure 1/3(Bc1_V)  "Bc1V"
  q1[rad]/1 -> [q1]  "q1"
  [q1] -> Structure 1/1(q1[rad])  "q1"
  q2[rad]/1 -> [q2]  "q2"
  [q2] -> Structure 2 (Revolute segment)/1(q2[rad])  "q2"
  Structure 1/2(PosVecs_S1) -> [PosVecsS1]  "PosVecs_S1"
  [PosVecsS1] -> Bus Creator4/1  "PosVecs_S1"
  Structure 2 (Revolute segment)/2(PosVecs_S2R) -> [PosVecsS2R]  "PosVecs_S2R"
  [PosVecsS2R] -> Bus Creator4/2  "PosVecs_S2R"
  [WRotXS2R] -> Bus Creator2/2  "WRotX_S2R"
  [WRotXS1] -> Bus Creator2/1  "WRotX_S1"
  [UMatS2R] -> Bus Creator/2  "UMats_S2R"
  [UMatS1] -> Bus Creator/1  "UMats_S1"
  [VelsS1] -> Bus Creator1/1  "Vels_S1"
  [VelsS2R] -> Bus Creator1/2  "Vels_S2R"
  [GeomS2R] -> Bus Creator3/2  "Geom_S2R"
  [GeomS1] -> Bus Creator3/1  "Geom_S1"
  Bus Creator3/1 -> [GeomSx]
  Bus Creator4/1 -> [PosVecsSx]
  Bus Creator2/1 -> [WRotXSx]
  Bus Creator1/1 -> [VelsSx]
  Bus Creator/1 -> [UMatSx]
  [GeomSx] -> GeomProp_Sx/1  "GeomSx"
  [PosVecsSx] -> PosVecs_Sx/1  "PosVecsSx"
  [WRotXSx] -> WRotX_Sx/1  "WRotSx"
  [VelsSx] -> Vels_Sx/1  "VelsSx"
  [UMatSx] -> UMat_Sx/1  "UMatSx"
  xt2[m]/1 -> [xt2]  "xt2"
  [xt2] -> Structure 2 (Prismatic segment)/1(xt2)  "xt2"
  [WRotXS2R] -> Structure 2 (Prismatic segment)/2(WRotX_S2R)  "WRotX_S2R"
  [VelsS2R] -> Structure 2 (Prismatic segment)/3(Vels_S2R)  "Vels_S2"
  Structure 2 (Prismatic segment)/1(GeomProp_S2P) -> [GeomS2P]  "Geom_S2P"
  [GeomS2P] -> Bus Creator3/3  "Geom_S2P"
  Structure 2 (Prismatic segment)/2(PosVecs_S2P) -> [PosVecsS2P]  "PosVecs_S2P"
  [PosVecsS2P] -> Bus Creator4/3  "PosVecs_S2P"
  Structure 2 (Prismatic segment)/3(WRotX_S2P) -> [WRotXS2P]  "WRotX_S2P"
  [WRotXS2P] -> Bus Creator2/3  "WRotX_S2P"
  Structure 2 (Prismatic segment)/4(Vels_S2P) -> [VelsS2P]  "Vels_S2P"
  Structure 2 (Prismatic segment)/5(UMats_S2P) -> [UMatsS2P]  "UMats_S2P"
  [UMatsS2P] -> Bus Creator/3  "UMats_S2P"
  [VelsS2P] -> Bus Creator1/3  "Vels_S2P"
  Bc1V/1 -> [Bc1V]  "Bc1V"

== system SimForcesGP2017a/Hydraulic manipulator, calculation/AngleRelations ==
  note: Pass to outputs...
  note: Process data...
  note: Get inputs...
  note: Calculate q1 and q2 from Theta1 and Theta2...
  Theta1[rad] : Inport
  Theta2[rad] : Inport  Port=2
  Fcn : Fcn  Expr=-pi/2 - beta1 - beta2 + u
  Fcn1 : Fcn  Expr=+u - beta3 - beta4
  q1[rad] : Outport
  q2[rad] : Outport  Port=2
  wires:
  Theta1[rad]/1 -> [Theta1]
  Theta2[rad]/1 -> [Theta2]
  [Theta2] -> Fcn1/1
  [Theta1] -> Fcn/1
  Fcn/1 -> [q1]
  [q1] -> q1[rad]/1
  [q2] -> q2[rad]/1
  Fcn1/1 -> [q2]

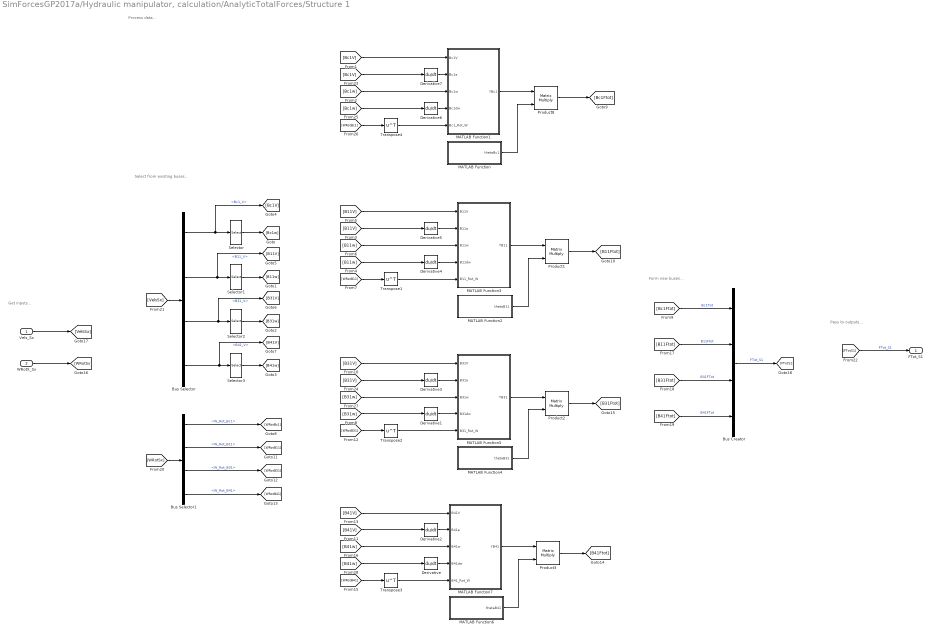
== system SimForcesGP2017a/Hydraulic manipulator, calculation/AnalyticTotalForces/Structure 1 ==
  note: Pass to outputs...
  note: Get inputs...
  note: Process data...
  note: Form new buses...
  note: Select from existing buses...
  Vels_Sx : Inport
  WRotX_Sx : Inport  Port=2
  Bus Creator : BusCreator  Inputs=Bc1Tot,B11Ftot,B31FTot,B41FTot
  Bus Selector : BusSelector  OutputSignals=Vels_S1.Bc1_V,Vels_S1.B11_V,Vels_S1.B31_V,Vels_S1.B41_V
  Bus Selector1 : BusSelector  OutputSignals=WRotX_S1.W_Rot_Bc1,WRotX_S1.W_Rot_B11,WRotX_S1.W_Rot_B31,WRotX_S1.W_Rot_B41
  Derivative{,1..7} (8 alike) : Derivative
  MATLAB Function : MATLAB Function  TreatAsAtomicUnit=on
  MATLAB Function1 : MATLAB Function  TreatAsAtomicUnit=on
  MATLAB Function2 : MATLAB Function  TreatAsAtomicUnit=on
  MATLAB Function3 : MATLAB Function  TreatAsAtomicUnit=on
  MATLAB Function4 : MATLAB Function  TreatAsAtomicUnit=on
  MATLAB Function5 : MATLAB Function  TreatAsAtomicUnit=on
  MATLAB Function6 : MATLAB Function  TreatAsAtomicUnit=on
  MATLAB Function7 : MATLAB Function  TreatAsAtomicUnit=on
  Product{1..3,8} (4 alike) : Product  Multiplication=Matrix(*)
  Selector{,1..3} (4 alike) : Selector  InputPortWidth=6  IndexOptions=Index vector (dialog)  Indices=[4 5 6]  OutputSizes=1
  Transpose{1..4} (4 alike) : Math  Operator=transpose  SignedPower=on  SaturateOnIntegerOverflow=on
  FTot_S1 : Outport
  wires:
  Bus Selector/4 -> Selector3/1, [B41V]  "<B41_V>"
  Bus Selector1/3 -> [WRotB31]  "<W_Rot_B31>"
  Bus Selector1/1 -> [WRotBc1]  "<W_Rot_Bc1>"
  [B11Ftot] -> Bus Creator/2  "B11Ftot"
  [WRotB31] -> Transpose2/1
  Selector/1 -> [Bc1w]
  Selector3/1 -> [B41w]
  Bus Selector/3 -> Selector2/1, [B31V]  "<B31_V>"
  [B31Ftot] -> Bus Creator/3  "B31FTot"
  Bus Selector/1 -> Selector/1, [Bc1V]  "<Bc1_V>"
  Bus Selector/2 -> Selector1/1, [B11V]  "<B11_V>"
  [B41Ftot] -> Bus Creator/4  "B41FTot"
  Selector2/1 -> [B31w]
  [Bc1Ftot] -> Bus Creator/1  "Bc1Tot"
  Bus Selector1/2 -> [WRotB11]  "<W_Rot_B11>"
  [WRotB11] -> Transpose1/1
  Bus Selector1/4 -> [WRotB41]  "<W_Rot_B41>"
  WRotX_Sx/1 -> [WRotSx]
  [WRotSx] -> Bus Selector1/1
  Vels_Sx/1 -> [VelsSx]
  [VelsSx] -> Bus Selector/1
  Bus Creator/1 -> [FTotS1]  "FTot_S1"
  [FTotS1] -> FTot_S1/1  "FTot_S1"
  Selector1/1 -> [B11w]
  [WRotBc1] -> Transpose4/1
  Transpose4/1 -> MATLAB Function1/5(Bc1_Rot_W)
  Derivative6/1 -> MATLAB Function1/4(Bc1dw)
  [Bc1w] -> Derivative6/1
  [Bc1V] -> Derivative7/1
  Derivative7/1 -> MATLAB Function1/2(Bc1a)
  MATLAB Function1/1(YBc1) -> Product8/1
  MATLAB Function/1(thetaBc1) -> Product8/2
  Product8/1 -> [Bc1Ftot]
  [Bc1V] -> MATLAB Function1/1(Bc1V)
  [Bc1w] -> MATLAB Function1/3(Bc1w)
  [B11w] -> MATLAB Function3/3(B11w)
  [B11V] -> MATLAB Function3/1(B11V)
  MATLAB Function2/1(thetaB11) -> Product1/2
  MATLAB Function3/1(YB11) -> Product1/1
  Derivative5/1 -> MATLAB Function3/2(B11a)
  [B11V] -> Derivative5/1
  [B11w] -> Derivative4/1
  Derivative4/1 -> MATLAB Function3/4(B11dw)
  Transpose1/1 -> MATLAB Function3/5(B11_Rot_W)
  Product1/1 -> [B11Ftot]
  Product2/1 -> [B31Ftot]
  Transpose2/1 -> MATLAB Function5/5(B31_Rot_W)
  Derivative1/1 -> MATLAB Function5/4(B31dw)
  [B31w] -> Derivative1/1
  [B31V] -> Derivative3/1
  Derivative3/1 -> MATLAB Function5/2(B31a)
  MATLAB Function5/1(YB31) -> Product2/1
  MATLAB Function4/1(thetaB31) -> Product2/2
  [B31V] -> MATLAB Function5/1(B31V)
  [B31w] -> MATLAB Function5/3(B31w)
  [B41w] -> MATLAB Function7/3(B41w)
  [B41V] -> MATLAB Function7/1(B41V)
  MATLAB Function6/1(thetaB41) -> Product3/2
  MATLAB Function7/1(YB41) -> Product3/1
  Derivative2/1 -> MATLAB Function7/2(B41a)
  [B41V] -> Derivative2/1
  [B41w] -> Derivative/1
  Derivative/1 -> MATLAB Function7/4(B41dw)
  Transpose3/1 -> MATLAB Function7/5(B41_Rot_W)
  Product3/1 -> [B41Ftot]
  [WRotB41] -> Transpose3/1

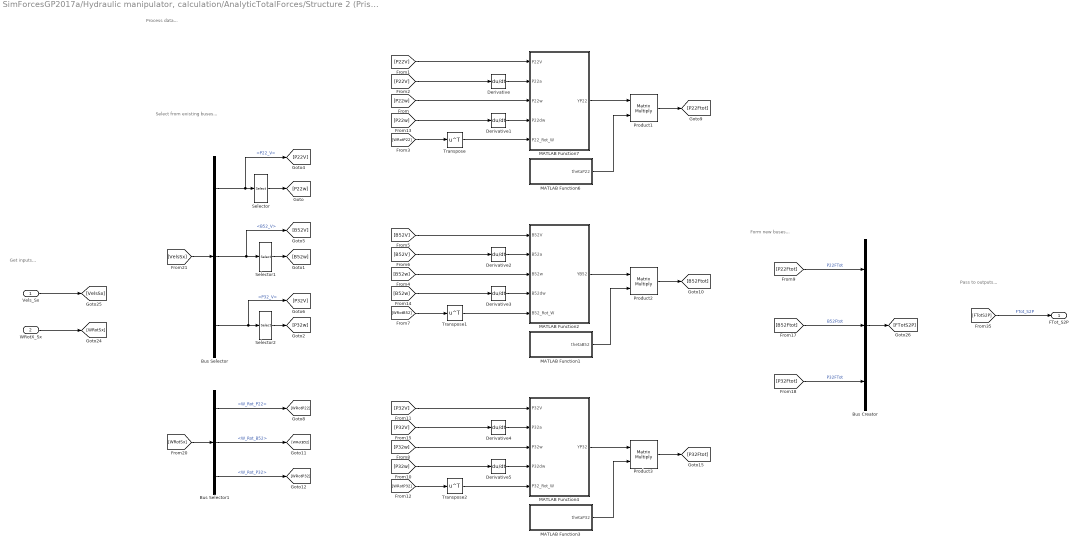
== system SimForcesGP2017a/Hydraulic manipulator, calculation/AnalyticTotalForces/Structure 2 (Prismatic segment) ==
  note: Select from existing buses...
  note: Form new buses...
  note: Get inputs...
  note: Pass to outputs...
  note: Process data...
  Vels_Sx : Inport
  WRotX_Sx : Inport  Port=2
  Bus Creator : BusCreator  Inputs=P22FTot,B52Ftot,P32FTot
  Bus Selector : BusSelector  OutputSignals=Vels_S2R.P22_V,Vels_S2P.B52_V,Vels_S2P.P32_V
  Bus Selector1 : BusSelector  OutputSignals=WRotX_S2R.W_Rot_P22,WRotX_S2P.W_Rot_B52,WRotX_S2P.W_Rot_P32
  Derivative{,1..5} (6 alike) : Derivative
  MATLAB Function1 : MATLAB Function  TreatAsAtomicUnit=on
  MATLAB Function2 : MATLAB Function  TreatAsAtomicUnit=on
  MATLAB Function3 : MATLAB Function  TreatAsAtomicUnit=on
  MATLAB Function4 : MATLAB Function  TreatAsAtomicUnit=on
  MATLAB Function6 : MATLAB Function  TreatAsAtomicUnit=on
  MATLAB Function7 : MATLAB Function  TreatAsAtomicUnit=on
  Product1 : Product  Multiplication=Matrix(*)
  Product2 : Product  Multiplication=Matrix(*)
  Product3 : Product  Multiplication=Matrix(*)
  Selector : Selector  InputPortWidth=6  IndexOptions=Index vector (dialog)  Indices=[4 5 6]  OutputSizes=1
  Selector1 : Selector  InputPortWidth=6  IndexOptions=Index vector (dialog)  Indices=[4 5 6]  OutputSizes=1
  Selector2 : Selector  InputPortWidth=6  IndexOptions=Index vector (dialog)  Indices=[4 5 6]  OutputSizes=1
  Transpose : Math  Operator=transpose  SignedPower=on  SaturateOnIntegerOverflow=on
  Transpose1 : Math  Operator=transpose  SignedPower=on  SaturateOnIntegerOverflow=on
  Transpose2 : Math  Operator=transpose  SignedPower=on  SaturateOnIntegerOverflow=on
  FTot_S2P : Outport
  wires:
  [FTotS2P] -> FTot_S2P/1  "FTot_S2P"
  WRotX_Sx/1 -> [WRotSx]
  Vels_Sx/1 -> [VelsSx]
  Product3/1 -> [P32Ftot]
  Bus Selector1/3 -> [WRotP32]  "<W_Rot_P32>"
  [VelsSx] -> Bus Selector/1
  Product2/1 -> [B52Ftot]
  Bus Selector1/1 -> [WRotP22]  "<W_Rot_P22>"
  [B52Ftot] -> Bus Creator/2  "B52Ftot"
  Product1/1 -> [P22Ftot]
  [WRotP22] -> Transpose/1
  [WRotP32] -> Transpose2/1
  Selector/1 -> [P22w]
  Bus Creator/1 -> [FTotS2P]
  [WRotSx] -> Bus Selector1/1
  Selector1/1 -> [B52w]
  [P32Ftot] -> Bus Creator/3  "P32FTot"
  Selector2/1 -> [P32w]
  [P22Ftot] -> Bus Creator/1  "P22FTot"
  Bus Selector1/2 -> [WRotB52]  "<W_Rot_B52>"
  Bus Selector/1 -> [P22V], Selector/1  "<P22_V>"
  Bus Selector/3 -> [P32V], Selector2/1  "<P32_V>"
  Bus Selector/2 -> [B52V], Selector1/1  "<B52_V>"
  [P22V] -> MATLAB Function7/1(P22V)
  Transpose/1 -> MATLAB Function7/5(P22_Rot_W)
  [P22V] -> Derivative/1
  [P22w] -> Derivative1/1
  MATLAB Function7/1(YP22) -> Product1/1
  Derivative1/1 -> MATLAB Function7/4(P22dw)
  MATLAB Function6/1(thetaP22) -> Product1/2
  Derivative/1 -> MATLAB Function7/2(P22a)
  [P22w] -> MATLAB Function7/3(P22w)
  MATLAB Function1/1(thetaB52) -> Product2/2
  MATLAB Function2/1(YB52) -> Product2/1
  [WRotB52] -> Transpose1/1
  [B52V] -> MATLAB Function2/1(B52V)
  [B52V] -> Derivative2/1
  Derivative2/1 -> MATLAB Function2/2(B52a)
  [B52w] -> MATLAB Function2/3(B52w)
  [B52w] -> Derivative3/1
  Derivative3/1 -> MATLAB Function2/4(B52dw)
  Transpose1/1 -> MATLAB Function2/5(B52_Rot_W)
  Transpose2/1 -> MATLAB Function4/5(P32_Rot_W)
  Derivative5/1 -> MATLAB Function4/4(P32dw)
  [P32w] -> Derivative5/1
  [P32w] -> MATLAB Function4/3(P32w)
  Derivative4/1 -> MATLAB Function4/2(P32a)
  [P32V] -> Derivative4/1
  [P32V] -> MATLAB Function4/1(P32V)
  MATLAB Function4/1(YP32) -> Product3/1
  MATLAB Function3/1(thetaP32) -> Product3/2

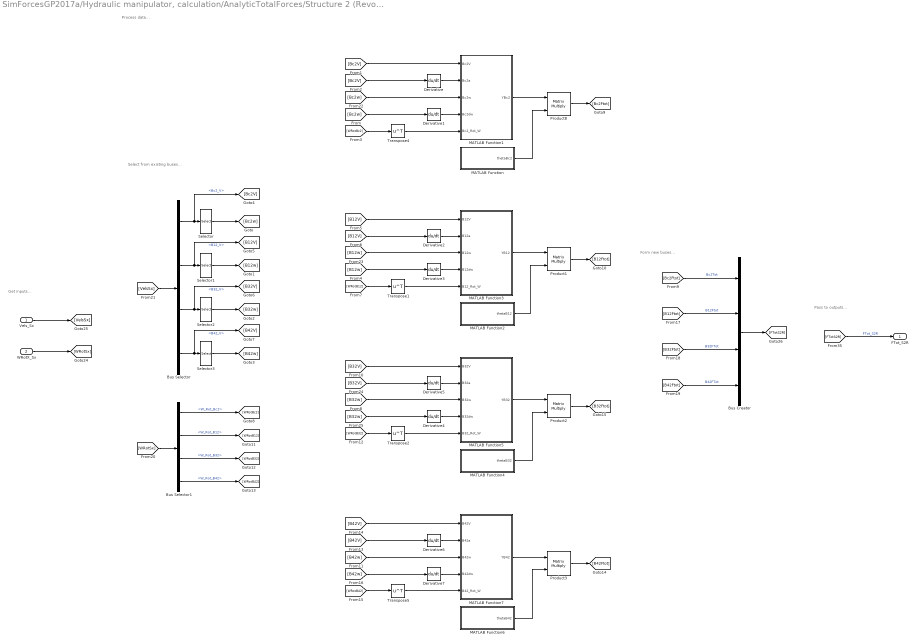
== system SimForcesGP2017a/Hydraulic manipulator, calculation/AnalyticTotalForces/Structure 2 (Revolute segment) ==
  note: Process data...
  note: Pass to outputs...
  note: Get inputs...
  note: Form new buses...
  note: Select from existing buses...
  Vels_Sx : Inport
  WRotX_Sx : Inport  Port=2
  Bus Creator : BusCreator  Inputs=Bc2Tot,B12Ftot,B32FTot,B42FTot
  Bus Selector : BusSelector  OutputSignals=Vels_S1.Bc2_V,Vels_S2R.B12_V,Vels_S2R.B32_V,Vels_S2R.B42_V
  Bus Selector1 : BusSelector  OutputSignals=WRotX_S1.W_Rot_Bc2,WRotX_S2R.W_Rot_B12,WRotX_S2R.W_Rot_B32,WRotX_S2R.W_Rot_B42
  Derivative{,1..7} (8 alike) : Derivative
  MATLAB Function : MATLAB Function  TreatAsAtomicUnit=on
  MATLAB Function1 : MATLAB Function  TreatAsAtomicUnit=on
  MATLAB Function2 : MATLAB Function  TreatAsAtomicUnit=on
  MATLAB Function3 : MATLAB Function  TreatAsAtomicUnit=on
  MATLAB Function4 : MATLAB Function  TreatAsAtomicUnit=on
  MATLAB Function5 : MATLAB Function  TreatAsAtomicUnit=on
  MATLAB Function6 : MATLAB Function  TreatAsAtomicUnit=on
  MATLAB Function7 : MATLAB Function  TreatAsAtomicUnit=on
  Product{1..3,8} (4 alike) : Product  Multiplication=Matrix(*)
  Selector{,1..3} (4 alike) : Selector  InputPortWidth=6  IndexOptions=Index vector (dialog)  Indices=[4 5 6]  OutputSizes=1
  Transpose{1..2,4..5} (4 alike) : Math  Operator=transpose  SignedPower=on  SaturateOnIntegerOverflow=on
  FTot_S2R : Outport
  wires:
  Bus Selector1/4 -> [WRotB42]  "<W_Rot_B42>"
  [WRotB12] -> Transpose1/1
  Bus Selector1/2 -> [WRotB12]  "<W_Rot_B12>"
  [WRotB42] -> Transpose5/1
  [Bc2Ftot] -> Bus Creator/1  "Bc2Tot"
  Selector2/1 -> [B32w]
  [B42Ftot] -> Bus Creator/4  "B42FTot"
  Bus Selector/2 -> Selector1/1, [B12V]  "<B12_V>"
  Bus Selector/1 -> Selector/1, [Bc2V]  "<Bc2_V>"
  [B32Ftot] -> Bus Creator/3  "B32FTot"
  Bus Selector/3 -> Selector2/1, [B32V]  "<B32_V>"
  Selector1/1 -> [B12w]
  [WRotSx] -> Bus Selector1/1
  Selector3/1 -> [B42w]
  Bus Creator/1 -> [FTotS2R]
  Selector/1 -> [Bc2w]
  [WRotB32] -> Transpose2/1
  Product3/1 -> [B42Ftot]
  Product8/1 -> [Bc2Ftot]
  [B12Ftot] -> Bus Creator/2  "B12Ftot"
  Bus Selector1/1 -> [WRotBc2]  "<W_Rot_Bc2>"
  [VelsSx] -> Bus Selector/1
  Bus Selector1/3 -> [WRotB32]  "<W_Rot_B32>"
  Bus Selector/4 -> Selector3/1, [B42V]  "<B42_V>"
  Vels_Sx/1 -> [VelsSx]
  WRotX_Sx/1 -> [WRotSx]
  [FTotS2R] -> FTot_S2R/1  "FTot_S2R"
  [Bc2w] -> Derivative1/1
  [Bc2w] -> MATLAB Function1/3(Bc2w)
  [WRotBc2] -> Transpose4/1
  Transpose4/1 -> MATLAB Function1/5(Bc2_Rot_W)
  Derivative1/1 -> MATLAB Function1/4(Bc2dw)
  [Bc2V] -> MATLAB Function1/1(Bc2V)
  MATLAB Function/1(thetaBc2) -> Product8/2
  [Bc2V] -> Derivative/1
  MATLAB Function1/1(YBc2) -> Product8/1
  Derivative/1 -> MATLAB Function1/2(Bc2a)
  Derivative2/1 -> MATLAB Function3/2(B12a)
  MATLAB Function3/1(YB12) -> Product1/1
  [B12V] -> Derivative2/1
  MATLAB Function2/1(thetaB12) -> Product1/2
  [B12V] -> MATLAB Function3/1(B12V)
  Derivative3/1 -> MATLAB Function3/4(B12dw)
  Transpose1/1 -> MATLAB Function3/5(B12_Rot_W)
  [B12w] -> MATLAB Function3/3(B12w)
  [B12w] -> Derivative3/1
  Product1/1 -> [B12Ftot]
  [B32w] -> Derivative4/1
  [B32w] -> MATLAB Function5/3(B32w)
  Derivative4/1 -> MATLAB Function5/4(B32dw)
  [B32V] -> MATLAB Function5/1(B32V)
  MATLAB Function4/1(thetaB32) -> Product2/2
  [B32V] -> Derivative5/1
  MATLAB Function5/1(YB32) -> Product2/1
  Derivative5/1 -> MATLAB Function5/2(B32a)
  Transpose2/1 -> MATLAB Function5/5(B32_Rot_W)
  Product2/1 -> [B32Ftot]
  Transpose5/1 -> MATLAB Function7/5(B42_Rot_W)
  Derivative6/1 -> MATLAB Function7/2(B42a)
  MATLAB Function7/1(YB42) -> Product3/1
  [B42V] -> Derivative6/1
  MATLAB Function6/1(thetaB42) -> Product3/2
  [B42V] -> MATLAB Function7/1(B42V)
  Derivative7/1 -> MATLAB Function7/4(B42dw)
  [B42w] -> MATLAB Function7/3(B42w)
  [B42w] -> Derivative7/1

== system SimForcesGP2017a/Hydraulic manipulator, calculation/AnalyticVelocities/Structure 1 ==
  note: Pass to outputs...
  note: Process data...
  note: Calculate geometric properties of the closed kinematic chain 1...
  note: Get inputs...
  note: Form relevant position vectors...
  note: Form relevant rotation matrices...
  note: Form relevant velocity/force transformation matrices...
  note: Form relevant linear/angular velocities...
  q1[rad] : Inport  Unit=rad
  W_Rot_Bc1 : Inport  Port=2
  Bc1_V : Inport  Port=3  PortDimensions=[6 1]
  GeomPropS1 : Subsystem
  PosVecsS1 : Subsystem
  RotMatsS1 : Subsystem
  UMatsS1 : Subsystem
  VelsS1 : Subsystem
  Geom_S1 : Outport
  PosVecs_S1 : Outport  Port=2
  WRotX_S1 : Outport  Port=3
  Vels_S1 : Outport  Port=4
  UMat_S1 : Outport  Port=5
  wires:
  GeomPropS1/1(GeomProp_S1) -> [GeomS1]
  [GeomS1] -> PosVecsS1/1(GeomProp_CC1)
  [GeomS1] -> RotMatsS1/1(GeomProp_S1)
  [GeomS1] -> VelsS1/1(GeomProp_S1)
  RotMatsS1/1(RotMats_S1) -> [RotMatsS1]
  [RotMatsS1] -> UMatsS1/2(RotMats_S1)
  PosVecsS1/1(PosVecs_S1) -> [PosVecsS1]
  [PosVecsS1] -> UMatsS1/1(PosVecs_S1)
  [GeomS1] -> Geom_S1/1
  VelsS1/1(Vels_S1) -> [VelsS1]
  [VelsS1] -> Vels_S1/1
  UMatsS1/1(UMat_S1) -> [UMatsS1]
  [UMatsS1] -> VelsS1/2(UMats_S1)
  Bc1_V/1 -> [Bc1V]  "Bc1V"
  [Bc1V] -> VelsS1/3(Bc1_V)
  W_Rot_Bc1/1 -> [WRotBc1]  "WRotBc1"
  [WRotBc1] -> RotMatsS1/2(WRotBc1)
  [UMatsS1] -> UMat_S1/1
  RotMatsS1/2(WRotX_S1) -> [WRotXS1]
  [WRotXS1] -> WRotX_S1/1
  q1[rad]/1 -> [q1]  "q1"
  [q1] -> GeomPropS1/1(q1)
  [PosVecsS1] -> PosVecs_S1/1

== system SimForcesGP2017a/Hydraulic manipulator, calculation/AnalyticVelocities/Structure 2 (Prismatic segment) ==
  note: Pass to outputs...
  note: Get inputs...
  note: Process data...
  xt2 : Inport
  WRotX_S2R : Inport  Port=2
  Vels_S2R : Inport  Port=3
  GeomPropS2P : Subsystem
  PosVecsS2P : Subsystem
  RotMatsS2P : Subsystem
  UMatsS2P : Subsystem
  VelsS2P : Subsystem
  GeomProp_S2P : Outport
  PosVecs_S2P : Outport  Port=2
  WRotX_S2P : Outport  Port=3
  Vels_S2P : Outport  Port=4
  UMats_S2P : Outport  Port=5
  wires:
  xt2/1 -> [xt2]
  Vels_S2R/1 -> [VelsS2R]
  WRotX_S2R/1 -> [WRotXS2R]
  GeomPropS2P/1(GeomProp_S2P) -> [GeomS2P]
  [GeomS2P] -> GeomProp_S2P/1
  [xt2] -> GeomPropS2P/1(xt2)
  PosVecsS2P/1(PosVecsS2P) -> [PosVecsS2P]
  [xt2] -> PosVecsS2P/1(xt2)
  [PosVecsS2P] -> PosVecs_S2P/1
  RotMatsS2P/2(WRotX_S2P) -> [WRotXS2P]
  [WRotXS2R] -> RotMatsS2P/1(WRotX_S2R)
  [WRotXS2P] -> WRotX_S2P/1
  RotMatsS2P/1(RotMats_S2P) -> [RotMatsS2P]
  [PosVecsS2P] -> UMatsS2P/1(PosVecs_S2P)
  [RotMatsS2P] -> UMatsS2P/2(RotMats_S2P)
  UMatsS2P/1(UMats_S2P) -> [UMatsS2P]
  [UMatsS2P] -> UMats_S2P/1
  [VelsS2R] -> VelsS2P/3(Vels_S2R)
  [GeomS2P] -> VelsS2P/1(GeomProp_S2P)
  [UMatsS2P] -> VelsS2P/2(UMats_S2P)
  VelsS2P/1(Vels_S2P) -> [VelsS2P]
  [VelsS2P] -> Vels_S2P/1

== system SimForcesGP2017a/Hydraulic manipulator, calculation/AnalyticVelocities/Structure 2 (Revolute segment) ==
  note: Pass to outputs...
  note: Process data...
  note: Get inputs...
  q2[rad] : Inport
  WRotX_S1 : Inport  Port=2
  Vels_S1 : Inport  Port=3
  GeomPropS2R : Subsystem
  PosVecsS2R : Subsystem
  RotMatsS2R : Subsystem
  UMatS2R : Subsystem
  VelsS2R : Subsystem
  GeomProp_S2R : Outport
  PosVecs_S2R : Outport  Port=2
  WRotX_S2R : Outport  Port=3
  Vels_S2R : Outport  Port=4
  UMats_S2R : Outport  Port=5
  wires:
  [GeomS2R] -> VelsS2R/1(GeomProp_CC2)
  [GeomS2R] -> RotMatsS2R/1(GeomProp_CC2)
  [GeomS2R] -> PosVecsS2R/1(GeomProp_S2R)
  GeomPropS2R/1(GeomProp_S2R) -> [GeomS2R]
  [q2] -> GeomPropS2R/1(q2)
  [GeomS2R] -> GeomProp_S2R/1  "GeomS2R"
  RotMatsS2R/1(RotMats_S2) -> [RotMatsS2R]
  q2[rad]/1 -> [q2]  "q2"
  PosVecsS2R/1(PosVecs_S2) -> [PosVecsS2R]
  [PosVecsS2R] -> UMatS2R/1(PosVecs_S2)
  [PosVecsS2R] -> PosVecs_S2R/1  "PosVecsS2R"
  [RotMatsS2R] -> UMatS2R/2(RotMats_S2)
  UMatS2R/1(UMatS2) -> [UMatsS2R]
  [UMatsS2R] -> VelsS2R/2(UMats_S2)
  [UMatsS2R] -> UMats_S2R/1  "UMatsS2R"
  RotMatsS2R/2(WRotX_S2) -> [WRotXS2R]
  [WRotXS2R] -> WRotX_S2R/1  "WRotXS2R"
  Vels_S1/1 -> [VelsS1]  "Vels_S1"
  [VelsS1] -> VelsS2R/3(Vels_S1)
  WRotX_S1/1 -> [WRotXS1]  "WRotX_S1"
  [WRotXS1] -> RotMatsS2R/2(WRotX_S1)
  VelsS2R/1(Vels_S2) -> [VelsS2R]
  [VelsS2R] -> Vels_S2R/1  "VelsS2R"
